simulink model "dcMotorSimulation"  (R2014a)
settings: Solver=ode45  StartTime=0.0  StopTime=10.0  RelTol=1e-3
libraries: simulink x1
settings Model: Creator=megaman  LastModifiedBy=megaman

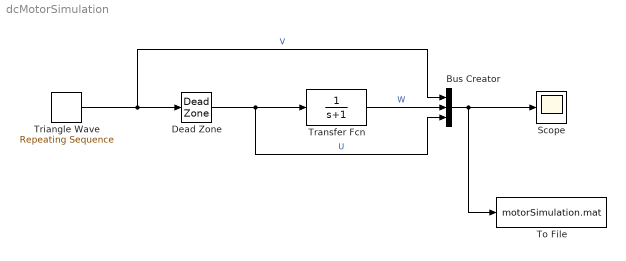
== system dcMotorSimulation ==
  Bus Creator : BusCreator  Inputs=3
  Dead Zone : DeadZone  UpperValue=0.6  SaturateOnIntegerOverflow=on
  Scope : Scope
  To File : ToFile  Filename=motorSimulation.mat  MatrixName=expData  SaveFormat=Timeseries
  Transfer Fcn : TransferFcn  Denominator=[1 1]
  Triangle Wave : simulink/Sources/Repeating Sequence  rep_seq_t=[0 1 2 3 4]  rep_seq_y=[0 1 0 -1 0]
  wires:
  Dead Zone/1 -> Transfer Fcn/1, Bus Creator/3  "U"
  Transfer Fcn/1 -> Bus Creator/2  "W"
  Triangle Wave/1 -> Bus Creator/1, Dead Zone/1  "V"
  Bus Creator/1 -> To File/1, Scope/1
